simulink model "ssg_speader_r1"  (Simulink 7.6)
settings: Solver=ode45  StartTime=0.0  StopTime=128000  RelTol=1e-3
undefined symbols (not defined in the file): ROACH
libraries: xbsIndex_r4 x1066, xps_library x48, casper_library_misc x28, dspsigops x16, simulink x8
(part 1 of 11)
settings Model: Creator=mwagner  LastModifiedBy=mwagner
settings DebuggingCC: StrictBusMsg=Warning

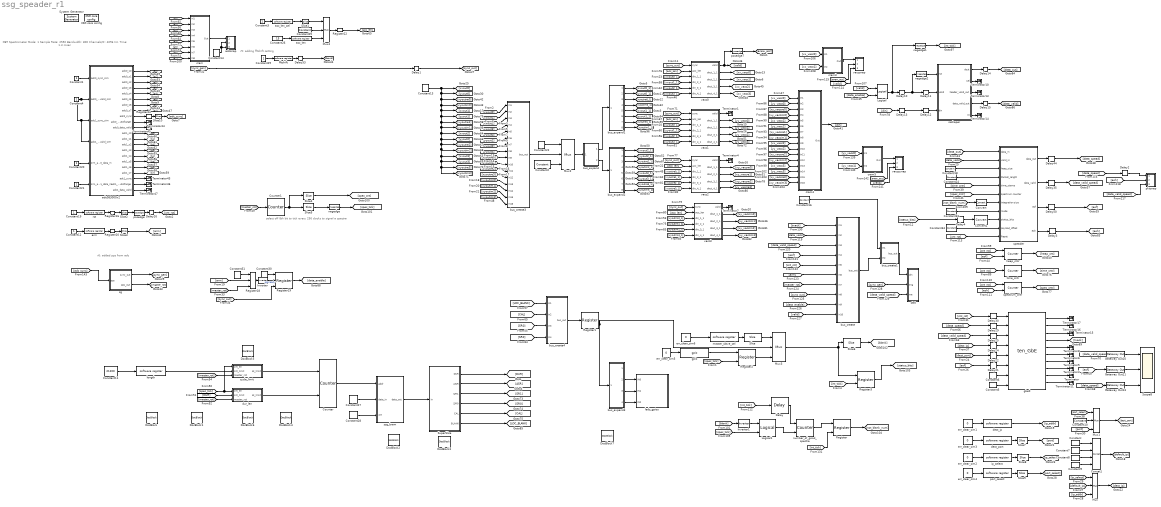
== system ssg_speader_r1 ==
  note: GBT Spectrometer
      | Mode: 1
      | Sample Rate: 2550
      | Bandwidth: 800
      | Channels/IF: 4096
      | Int. Time: 1.3 msec
  note: r5: adding fftshift setting
  note: r6: added pps from adc
  note: select off 8th bit to tick every 256 clocks to signal a spectra
  " System Generator" : xbsIndex_r4/ System Generator  Tag=genX  SystemSampleTime=-1  xilinxfamily=virtex5  part=xc5vsx95t  speed=-1  package=ff1136  synthesis_tool=XST  clock_wrapper=Clock Enables  directory=./vegas01_4tap_1024ch_220_r5a/sysgen  proj_type=Project Navigator  Synth_file=XST Defaults  Impl_file=ISE Defaults  testbench=off  simulink_period=1  sysclk_period=6.6667  dcm_input_clock_period=100  incr_netlist=off  trim_vbits=Everywhere in SubSystem  dbl_ovrd=According to Block Masks  core_generation=According to Block Masks  run_coregen=off  deprecated_control=off  eval_field=0  block_type=sysgen
      settings: block_version=10.1.3
  Concat1 : xbsIndex_r4/Concat  num_inputs=4  dbl_ovrd=off  block_type=concat
  Constant : xbsIndex_r4/Constant  const=10  gui_display_data_type=Fixed-point  arith_type=Unsigned  n_bits=8  bin_pt=0  preci_type=Single  exp_width=8  frac_width=24  explicit_period=on  period=1  equ=P=C  opselect=C  inp2=PCIN>>17  opr=+  inp1=P  carry=CIN  dbl_ovrd=off  block_type=constant
      settings: block_version=11.4
  Constant{1,4,20..21} (4 alike) : Constant  SampleTime=1
  Constant10 : xbsIndex_r4/Constant  const=10145  gui_display_data_type=Fixed-point  arith_type=Unsigned  n_bits=32  bin_pt=0  preci_type=Single  exp_width=8  frac_width=24  explicit_period=on  period=1  equ=P=C  opselect=C  inp2=PCIN>>17  opr=+  inp1=P  carry=CIN  dbl_ovrd=off  block_type=constant
  Constant11 : Constant  Value=21200  VectorParams1D=off
  Constant{3,12,19,29} (4 alike) : Constant
  Constant13 : xbsIndex_r4/Constant  const=1  gui_display_data_type=Fixed-point  arith_type=Unsigned  n_bits=32  bin_pt=0  preci_type=Single  exp_width=8  frac_width=24  explicit_period=on  period=1  equ=P=C  opselect=C  inp2=PCIN>>17  opr=+  inp1=P  carry=CIN  dbl_ovrd=off  block_type=constant
      settings: block_version=11.4
  Constant14 : xbsIndex_r4/Constant  const=1  gui_display_data_type=Fixed-point  arith_type=Boolean  n_bits=16  bin_pt=0  preci_type=Single  exp_width=8  frac_width=24  explicit_period=on  period=1  equ=P=C  opselect=C  inp2=PCIN>>17  opr=+  inp1=P  carry=CIN  dbl_ovrd=off  block_type=constant
      settings: block_version=11.4
  Constant16 : xbsIndex_r4/Constant  const=0  gui_display_data_type=Fixed-point  arith_type=Unsigned  n_bits=32-10  bin_pt=0  preci_type=Single  exp_width=8  frac_width=24  explicit_period=on  period=1  equ=P=C  opselect=C  inp2=PCIN>>17  opr=+  inp1=P  carry=CIN  dbl_ovrd=off  block_type=constant
  Constant18 : xbsIndex_r4/Constant  const=16384+8*6  gui_display_data_type=Fixed-point  arith_type=Unsigned  n_bits=40  bin_pt=0  preci_type=Single  exp_width=8  frac_width=24  explicit_period=on  period=1  equ=P=C  opselect=C  inp2=PCIN>>17  opr=+  inp1=P  carry=CIN  dbl_ovrd=off  block_type=constant
  Constant2 : xbsIndex_r4/Constant  const=0  gui_display_data_type=Fixed-point  arith_type=Unsigned  n_bits=512  bin_pt=0  preci_type=Single  exp_width=8  frac_width=24  explicit_period=on  period=1  equ=P=C  opselect=C  inp2=PCIN>>17  opr=+  inp1=P  carry=CIN  dbl_ovrd=off  block_type=constant
  Constant22 : xbsIndex_r4/Constant  const=0  gui_display_data_type=Boolean  arith_type=Boolean  n_bits=16  bin_pt=0  preci_type=Single  exp_width=8  frac_width=24  explicit_period=on  period=1  equ=P=C  opselect=C  inp2=PCIN>>17  opr=+  inp1=P  carry=CIN  dbl_ovrd=off  block_type=constant
      settings: block_version=11.4
  Constant24 : xbsIndex_r4/Constant  const=8192  gui_display_data_type=Fixed-point  arith_type=Unsigned  n_bits=40  bin_pt=0  preci_type=Single  exp_width=8  frac_width=24  explicit_period=on  period=1  equ=P=C  opselect=C  inp2=PCIN>>17  opr=+  inp1=P  carry=CIN  dbl_ovrd=off  block_type=constant
  Constant25 : xbsIndex_r4/Constant  const=63  gui_display_data_type=Fixed-point  arith_type=Unsigned  n_bits=32  bin_pt=0  preci_type=Single  exp_width=8  frac_width=24  explicit_period=on  period=1  equ=P=C  opselect=C  inp2=PCIN>>17  opr=+  inp1=P  carry=CIN  dbl_ovrd=off  block_type=constant
  Constant26 : Constant  Value=15
  Constant27 : xbsIndex_r4/Constant  const=0  gui_display_data_type=Fixed-point  arith_type=Unsigned  n_bits=32  bin_pt=0  preci_type=Single  exp_width=8  frac_width=24  explicit_period=on  period=1  equ=P=C  opselect=C  inp2=PCIN>>17  opr=+  inp1=P  carry=CIN  dbl_ovrd=off  block_type=constant
      settings: block_version=11.3
  Constant28 : xbsIndex_r4/Constant  const=0  gui_display_data_type=Fixed-point  arith_type=Boolean  n_bits=32  bin_pt=0  preci_type=Single  exp_width=8  frac_width=24  explicit_period=on  period=1  equ=P=C  opselect=C  inp2=PCIN>>17  opr=+  inp1=P  carry=CIN  dbl_ovrd=off  block_type=constant
      settings: block_version=11.3
  Constant30 : xbsIndex_r4/Constant  const=1  gui_display_data_type=Fixed-point  arith_type=Boolean  n_bits=16  bin_pt=0  preci_type=Single  exp_width=8  frac_width=24  explicit_period=on  period=1  equ=P=C  opselect=C  inp2=PCIN>>17  opr=+  inp1=P  carry=CIN  dbl_ovrd=off  block_type=constant
      settings: block_version=11.4
  Constant31 : xbsIndex_r4/Constant  const=1  gui_display_data_type=Fixed-point  arith_type=Boolean  n_bits=16  bin_pt=0  preci_type=Single  exp_width=8  frac_width=24  explicit_period=on  period=1  equ=P=C  opselect=C  inp2=PCIN>>17  opr=+  inp1=P  carry=CIN  dbl_ovrd=off  block_type=constant
      settings: block_version=11.4
  Constant33 : xbsIndex_r4/Constant  const=1  gui_display_data_type=Fixed-point  arith_type=Unsigned  n_bits=40  bin_pt=0  preci_type=Single  exp_width=8  frac_width=24  explicit_period=on  period=1  equ=P=C  opselect=C  inp2=PCIN>>17  opr=+  inp1=P  carry=CIN  dbl_ovrd=off  block_type=constant
  Constant34 : xbsIndex_r4/Constant  const=0  gui_display_data_type=Fixed-point  arith_type=Unsigned  n_bits=40  bin_pt=0  preci_type=Single  exp_width=8  frac_width=24  explicit_period=on  period=1  equ=P=C  opselect=C  inp2=PCIN>>17  opr=+  inp1=P  carry=CIN  dbl_ovrd=off  block_type=constant
  Constant5 : xbsIndex_r4/Constant  const=0  gui_display_data_type=Fixed-point  arith_type=Boolean  n_bits=1  bin_pt=0  preci_type=Single  exp_width=8  frac_width=24  explicit_period=on  period=1  equ=P=C  opselect=C  inp2=PCIN>>17  opr=+  inp1=P  carry=CIN  dbl_ovrd=off  block_type=constant
  Constant6 : xbsIndex_r4/Constant  const=0  gui_display_data_type=Fixed-point  arith_type=Boolean  n_bits=1  bin_pt=0  preci_type=Single  exp_width=8  frac_width=24  explicit_period=on  period=1  equ=P=C  opselect=C  inp2=PCIN>>17  opr=+  inp1=P  carry=CIN  dbl_ovrd=off  block_type=constant
  Constant7 : xbsIndex_r4/Constant  const=0  gui_display_data_type=Fixed-point  arith_type=Unsigned  n_bits=8  bin_pt=0  preci_type=Single  exp_width=8  frac_width=24  explicit_period=on  period=1  equ=P=C  opselect=C  inp2=PCIN>>17  opr=+  inp1=P  carry=CIN  dbl_ovrd=off  block_type=constant
      settings: block_version=11.4
  Constant8 : xbsIndex_r4/Constant  const=0  gui_display_data_type=Fixed-point  arith_type=Unsigned  n_bits=8  bin_pt=0  preci_type=Single  exp_width=8  frac_width=24  explicit_period=on  period=1  equ=P=C  opselect=C  inp2=PCIN>>17  opr=+  inp1=P  carry=CIN  dbl_ovrd=off  block_type=constant
      settings: block_version=11.4
  Constant9 : xbsIndex_r4/Constant  const=145  gui_display_data_type=Fixed-point  arith_type=Unsigned  n_bits=8  bin_pt=0  preci_type=Single  exp_width=8  frac_width=24  explicit_period=on  period=1  equ=P=C  opselect=C  inp2=PCIN>>17  opr=+  inp1=P  carry=CIN  dbl_ovrd=off  block_type=constant
      settings: block_version=11.4
  Convert : xbsIndex_r4/Convert  gui_display_data_type=Fixed-point  arith_type=Unsigned  n_bits=40  bin_pt=0  float_type=Single  exp_bits=8  fraction_bits=24  quantization=Truncate  overflow=Wrap  en=off  latency=0  dbl_ovrd=off  pipeline=off  block_type=convert
      settings: block_version=11.4
  Convert1 : xbsIndex_r4/Convert  gui_display_data_type=Fixed-point  arith_type=Unsigned  n_bits=40  bin_pt=0  float_type=Single  exp_bits=8  fraction_bits=24  quantization=Truncate  overflow=Wrap  en=off  latency=0  dbl_ovrd=off  pipeline=off  block_type=convert
  Counter : xbsIndex_r4/Counter  cnt_type=Free Running  cnt_to=Inf  operation=Up  start_count=0  cnt_by_val=1  arith_type=Unsigned  n_bits=8  bin_pt=0  load_pin=off  rst=on  en=on  explicit_period=on  period=1  dbl_ovrd=off  use_behavioral_HDL=off  implementation=DSP48  block_type=counter
      settings: block_version=11.3
  Counter1 : xbsIndex_r4/Counter  cnt_type=Free Running  cnt_to=Inf  operation=Up  start_count=0  cnt_by_val=1  arith_type=Unsigned  n_bits=48  bin_pt=0  load_pin=off  rst=on  en=off  explicit_period=on  period=1  dbl_ovrd=off  use_behavioral_HDL=off  implementation=DSP48  block_type=counter
      settings: block_version=11.3
  Delay : xbsIndex_r4/Delay  rst=off  infoeditControl=Selection of Reset will increase slice count due to use of real FFs and instead of SRLs  en=off  latency=1  dbl_ovrd=off  reg_retiming=off  block_type=delay
  Delay1 : xbsIndex_r4/Delay  rst=off  infoeditControl=Selection of Reset will increase slice count due to use of real FFs and instead of SRLs  en=off  latency=1000  dbl_ovrd=off  reg_retiming=off  block_type=delay
      settings: block_version=11.4
  Delay{10..13} (4 alike) : xbsIndex_r4/Delay  rst=off  infoeditControl=Selection of Reset will increase slice count due to use of real FFs and instead of SRLs  en=off  latency=2  dbl_ovrd=off  reg_retiming=on  block_type=delay
  Delay14 : xbsIndex_r4/Delay  rst=off  infoeditControl=Selection of Reset will increase slice count due to use of real FFs and instead of SRLs  en=off  latency=4  dbl_ovrd=off  reg_retiming=on  block_type=delay
  Delay15 : xbsIndex_r4/Delay  rst=off  infoeditControl=Selection of Reset will increase slice count due to use of real FFs and instead of SRLs  en=off  latency=4  dbl_ovrd=off  reg_retiming=on  block_type=delay
  Delay2 : xbsIndex_r4/Delay  rst=off  infoeditControl=Selection of Reset will increase slice count due to use of real FFs and instead of SRLs  en=off  latency=12  dbl_ovrd=off  reg_retiming=on  block_type=delay
  Delay{3..4,21..22,24..25,29..30,35,44,50} (11 alike) : xbsIndex_r4/Delay  rst=off  infoeditControl=Selection of Reset will increase slice count due to use of real FFs and instead of SRLs  en=off  latency=1  dbl_ovrd=off  reg_retiming=on  block_type=delay
  Delay26 : xbsIndex_r4/Delay  rst=off  infoeditControl=Selection of Reset will increase slice count due to use of real FFs and instead of SRLs  en=off  latency=8  dbl_ovrd=off  reg_retiming=on  block_type=delay
  Delay53 : xbsIndex_r4/Delay  rst=off  infoeditControl=Selection of Reset will increase slice count due to use of real FFs and instead of SRLs  en=off  latency=1  dbl_ovrd=off  reg_retiming=off  block_type=delay
      settings: block_version=11.4
  DocBlock{,1..7} (8 alike) : simulink/Model-Wide Utilities/DocBlock  SystemSampleTime=-1  DocumentType=Text
  Gateway Out10 : xbsIndex_r4/Gateway Out  hdl_port=on  timing_constraint=None  locs_specified=off  LOCs={}  block_type=gatewayout
      settings: infoedit="Gateway out block.  Converts Xilinx fixed point inputs into ouputs of type Simulink integer, double, or fixed point.<br><br>Hardware notes:  In hardware these blocks become top level output ports or are discarded, depending on how they are configured."  block_version=11.4
  Gateway Out11 : xbsIndex_r4/Gateway Out  hdl_port=on  timing_constraint=None  locs_specified=off  LOCs={}  block_type=gatewayout
      settings: infoedit="Gateway out block.  Converts Xilinx fixed point inputs into ouputs of type Simulink integer, double, or fixed point.<br><br>Hardware notes:  In hardware these blocks become top level output ports or are discarded, depending on how they are configured."  block_version=11.4
  Gateway Out13 : xbsIndex_r4/Gateway Out  hdl_port=on  timing_constraint=None  locs_specified=off  LOCs={}  block_type=gatewayout
      settings: infoedit="Gateway out block.  Converts Xilinx fixed point inputs into ouputs of type Simulink integer, double, or fixed point.<br><br>Hardware notes:  In hardware these blocks become top level output ports or are discarded, depending on how they are configured."  block_version=11.4
  Inverter : xbsIndex_r4/Inverter  en=off  latency=0  dbl_ovrd=off  block_type=inv
      settings: block_version=11.4
  Inverter1 : xbsIndex_r4/Inverter  en=off  latency=0  dbl_ovrd=off  block_type=inv
  Logical : xbsIndex_r4/Logical  logical_function=AND  inputs=2  en=off  latency=0  precision=Full  arith_type=Unsigned  n_bits=16  bin_pt=0  align_bp=on  dbl_ovrd=off  block_type=logical
      settings: block_version=11.4
  Logical1 : xbsIndex_r4/Logical  logical_function=AND  inputs=2  en=off  latency=0  precision=Full  arith_type=Unsigned  n_bits=16  bin_pt=0  align_bp=on  dbl_ovrd=off  block_type=logical
  Mux{,1..2,4} (4 alike) : xbsIndex_r4/Mux  inputs=2  en=off  latency=1  precision=Full  arith_type=Unsigned  n_bits=16  bin_pt=14  quantization=Truncate  overflow=Wrap  dbl_ovrd=off  block_type=mux
      Mux settings: block_version=11.4
      Mux1 settings: block_version=11.4
      Mux4 settings: block_version=11.4
  Mux3 : xbsIndex_r4/Mux  inputs=2  en=off  latency=0  precision=Full  arith_type=Unsigned  n_bits=16  bin_pt=14  quantization=Truncate  overflow=Wrap  dbl_ovrd=off  block_type=mux
  Register : xbsIndex_r4/Register  init=0  rst=off  en=on  dbl_ovrd=off  block_type=register
  Register{1,16,20,22,44} (5 alike) : xbsIndex_r4/Register  init=0  rst=off  en=off  dbl_ovrd=off  block_type=register
      settings: block_version=11.4
  Register18 : xbsIndex_r4/Register  init=0  rst=on  en=on  dbl_ovrd=off  block_type=register
      settings: block_version=11.4
  Register19 : xbsIndex_r4/Register  init=0  rst=on  en=on  dbl_ovrd=off  block_type=register
      settings: block_version=11.4
  Register2 : xbsIndex_r4/Register  init=0  rst=off  en=on  dbl_ovrd=off  block_type=register
      settings: block_version=11.4
  Register3 : xbsIndex_r4/Register  init=0  rst=off  en=on  dbl_ovrd=off  block_type=register
      settings: block_version=11.4
  Scope8 : Scope  NumInputPorts=3
      settings: TimeRange=4500  YMin=0~-1~0  YMax=1~1~1.75e+13  SaveName=ScopeData8  MaxDataPoints=100000
  Slice{,1..3,8..10} (7 alike) : xbsIndex_r4/Slice  nbits=1  boolean_output=on  mode=Lower Bit Location + Width  bit1=0  base1=MSB of Input  bit0=0  base0=LSB of Input  dbl_ovrd=off  block_type=slice
      Slice1 settings: block_version=10.1.3
      Slice10 settings: infoedit="Extracts a given range of bits from each input sample and presents it at the output.  The output type is ordinarily unsigned with binary point at zero, but can be Boolean when the slice is one bit wide.<P><P>Hardware notes: In hardware this block costs nothing."  block_version=10.1.3
      Slice2 settings: block_version=10.1.3
      Slice3 settings: block_version=10.1.3
      Slice8 settings: block_version=10.1.3
      Slice9 settings: block_version=10.1.3
  Slice4 : xbsIndex_r4/Slice  nbits=40  boolean_output=off  mode=Lower Bit Location + Width  bit1=0  base1=MSB of Input  bit0=8  base0=LSB of Input  dbl_ovrd=off  block_type=slice
      settings: block_version=10.1.3
  Slice5 : xbsIndex_r4/Slice  nbits=1  boolean_output=on  mode=Lower Bit Location + Width  bit1=7  base1=MSB of Input  bit0=7  base0=LSB of Input  dbl_ovrd=off  block_type=slice
      settings: block_version=10.1.3
  Slice6 : xbsIndex_r4/Slice  nbits=1  boolean_output=on  mode=Upper Bit Location + Width  bit1=0  base1=MSB of Input  bit0=0  base0=LSB of Input  dbl_ovrd=off  block_type=slice
  Slice7 : xbsIndex_r4/Slice  nbits=16  boolean_output=off  mode=Lower Bit Location + Width  bit1=0  base1=MSB of Input  bit0=0  base0=LSB of Input  dbl_ovrd=off  block_type=slice
      settings: infoedit="Extracts a given range of bits from each input sample and presents it at the output.  The output type is ordinarily unsigned with binary point at zero, but can be Boolean when the slice is one bit wide.<P><P>Hardware notes: In hardware this block costs nothing."  block_version=10.1.3
  SuperSlice : Subsystem  AncestorBlock=gavrt_library/SuperSlice  mask(superslice){slices=[27,1,1,1,1,1]}
      mask prompts: slices "Slice pattern"
      mask help:
      | Slices the input word into consecutive outputs of arbitrary width.
      | Slice pattern should be a vector with each entry representing the width of that particular slice. The first entry is the MSB slice and the last is the LSB slice.
      | If a slice is given width -1, that slice will have a boolean output.
      | Ex: -1*ones(1,32)  -- Slice a 32 bit word into seperate boolean flags
      | [16, 8, -1*ones(1,8)] -- Slice a 32 bit word into the MSW, a byte, and the least significant 8 bits
      mask init:
      | superslice_init(gcb, 'slices', slices);
  Terminator{,1,3..8,10..11,13..17,43..47} (20 alike) : Terminator
  XSG core config : xps_library/XSG core config  Tag=xps:xsg  SystemSampleTime=-1  hw_sys=ROACH:sx95t  ibob_linux=off  clk_src=adc0_clk  iBOB_clk_src=adc0_clk  BEE2_ctrl_clk_src=sys_clk  BEE2_usr_clk_src=sys_clk  ROACH_clk_src=adc0_clk  ROACH2_clk_src=adc0_clk  CORR_clk_src=sys_clk  gpio_clk_io_group=iBOB:sma  gpio_clk_bit_index=0  clk_rate=150  sample_period=1  synthesis_tool=XST  mpc_type=powerpc440_ext
  acc_len : xps_library/software register  Tag=xps:sw_reg  SystemSampleTime=-1  io_dir=From Processor  arith_type=Unsigned  bitwidth=32  bin_pt=0  sample_period=1  gw_name=ssg_speader_crash_acc_len_user_data_out
      link override convert: arith_type=Unsigned  n_bits=32  bin_pt=0
      link override r_spec_2048_r102_cnt_rst_user_data_out: arith_type=Unsigned  n_bits=32  bin_pt=0  period=1
      link override r_spec_2048_r102_nosim_cnt_rst_user_data_out: arith_type=Unsigned  n_bits=32  bin_pt=0  period=1
      link override r_spec_2048_r103_cnt_rst_user_data_out: arith_type=Unsigned  n_bits=32  bin_pt=0  period=1
      link override roach_spec_no10gbe_sync_cnt_rst_user_data_out: arith_type=Unsigned  n_bits=32  bin_pt=0  period=1
      link override roach_spec_rst_cnt_user_data_out: arith_type=Unsigned  n_bits=32  bin_pt=0  period=1
      link override roach_spec_rst_sync_cnt_user_data_out: arith_type=Unsigned  n_bits=32  bin_pt=0  period=1
  acc_len_sel : xps_library/software register  Tag=xps:sw_reg  SystemSampleTime=-1  io_dir=From Processor  arith_type=Unsigned  bitwidth=32  bin_pt=0  sample_period=1  gw_name=ssg_speader_crash_acc_len_sel_user_data_out
      link override convert: arith_type=Unsigned  n_bits=32  bin_pt=0
      link override r_spec_2048_r102_cnt_rst_user_data_out: arith_type=Unsigned  n_bits=32  bin_pt=0  period=1
      link override r_spec_2048_r102_nosim_cnt_rst_user_data_out: arith_type=Unsigned  n_bits=32  bin_pt=0  period=1
      link override r_spec_2048_r103_cnt_rst_user_data_out: arith_type=Unsigned  n_bits=32  bin_pt=0  period=1
      link override roach_spec_no10gbe_sync_cnt_rst_user_data_out: arith_type=Unsigned  n_bits=32  bin_pt=0  period=1
      link override roach_spec_rst_cnt_user_data_out: arith_type=Unsigned  n_bits=32  bin_pt=0  period=1
      link override roach_spec_rst_sync_cnt_user_data_out: arith_type=Unsigned  n_bits=32  bin_pt=0  period=1
  adc083000x2 : Subsystem  Tag=xps:adc083000x2  AncestorBlock=xps_library/adc083000x2  mask(adc_083000x2){use_adc0=on, use_adc1=on, demux_adc=off, clock_sync=off, verbose=off, using_ctrl=on, adc_clk_rate=600, sample_period=1, bit_width=8}
      mask prompts: use_adc0 "Use ZD0K0?"; use_adc1 "Use ZDOK1?"; demux_adc "Demux ADCs by 2?"; clock_sync "Interleave 2 ADC boards?"; verbose "Verbose Block Creation?"; using_ctrl "Add ports for control registers?"; adc_clk_rate "ADC clock rate (MHz)"; sample_period "Sample Period"; bit_width "Output Bit Width"
      mask help:
      | The ADC block converts analog inputs to digital outputs.
      | Every clock cycle, the inputs are sampled and digitized to
      | 8 bit binary point numbers in the range of [-1, 1).
      |
      | Online block-specific documentation: http://casper.berkeley.edu/wiki/Adc083000
      mask init:
      | adc083000_mask;
      mask Help: eval('xlWeb([getenv(''MLIB_ROOT''), ''\doc\html\sys_adc\sys_adc.html''])')
  adcsnap : Subsystem  AncestorBlock=casper_library_scopes/snap64  mask(snap64){nsamples=11}
      mask prompts: nsamples "No. of samples(2^?)"
      mask help:
      | The <i>snap</i> block provides a packaged solution to capturing data from
      | the FPGA fabric and making it accessible from the CPU.  The block comes in
      | 2 flavors: <i>snap</i> (which captures to a 32 bit wide Shared BRAM), and
      | <i>snap64</i> (which captures to 2x32 bit wide Shared BRAMs to effect a
      | 64 bit capture).
      mask Help: eval('xlWeb(''http://casper.berkeley.edu/wiki/Snap'')')
  arm : xps_library/software register  Tag=xps:sw_reg  SystemSampleTime=-1  io_dir=From Processor  arith_type=Unsigned  bitwidth=32  bin_pt=0  sample_period=1  gw_name=ssg_speader_crash_arm_user_data_out
      link override convert: arith_type=Unsigned  n_bits=32  bin_pt=0
      link override r_spec_2048_r102_cnt_rst_user_data_out: arith_type=Unsigned  n_bits=32  bin_pt=0  period=1
      link override r_spec_2048_r102_nosim_cnt_rst_user_data_out: arith_type=Unsigned  n_bits=32  bin_pt=0  period=1
      link override r_spec_2048_r103_cnt_rst_user_data_out: arith_type=Unsigned  n_bits=32  bin_pt=0  period=1
      link override roach_spec_no10gbe_sync_cnt_rst_user_data_out: arith_type=Unsigned  n_bits=32  bin_pt=0  period=1
      link override roach_spec_rst_cnt_user_data_out: arith_type=Unsigned  n_bits=32  bin_pt=0  period=1
      link override roach_spec_rst_sync_cnt_user_data_out: arith_type=Unsigned  n_bits=32  bin_pt=0  period=1
  bus_create : Subsystem  AncestorBlock=casper_library_flow_control/bus_create  mask(bus_create){inputNum=10}
      mask prompts: inputNum "Number of inputs:"
      mask init:
      | bus_create_init(gcb,...
      |     'inputNum', inputNum);
  bus_create1 : Subsystem  AncestorBlock=casper_library_flow_control/bus_create  mask(bus_create){inputNum=2}
      mask prompts: inputNum "Number of inputs:"
      mask init:
      | bus_create_init(gcb,...
      |     'inputNum', inputNum);
  bus_create3 : Subsystem  AncestorBlock=casper_library_flow_control/bus_create  mask(bus_create){inputNum=16}
      mask prompts: inputNum "Number of inputs:"
      mask init:
      | bus_create_init(gcb,...
      |     'inputNum', inputNum);
  bus_create4 : Subsystem  AncestorBlock=casper_library_flow_control/bus_create  mask(bus_create){inputNum=4}
      mask prompts: inputNum "Number of inputs:"
      mask init:
      | bus_create_init(gcb,...
      |     'inputNum', inputNum);
  bus_expand : Subsystem  AncestorBlock=casper_library_flow_control/bus_expand  mask(bus_expand){mode=divisions of equal size, outputNum=2, outputWidth=256, outputBinaryPt=0, outputArithmeticType=0, outputToWorkspace=off, variablePrefix=out, outputToModelAsWell=on}
      mask prompts: outputNum "Number of outputs:"; outputWidth "Output width:"; outputBinaryPt "Output binary point position:"; outputArithmeticType "Output arithmetic type: (Unsigned=0, Signed=1, Boolean=2)"; outputToWorkspace "Output to workspace?"; variablePrefix "Variable name prefix:"; outputToModelAsWell "Output to model as well?"
      mask help:
      | Expands a 'bus' made using a bus_create or Xilinx
      | concat block.
      | The input will be divided into the specified number
      | of outputs with the specified arithmetic types.
      | Divisions are made from most significant bit.
      mask init:
      | bus_expand_init(gcb,...
      |     'mode', mode, ...
      |     'outputNum', outputNum, ...
      |     'outputWidth', outputWidth, ...
      |     'outputBinaryPt', outputBinaryPt, ...
      |     'outputArithmeticType', outputArithmeticType, ...
      |     'outputToWorkspace', outputToWorkspace, ...
      |     'variablePrefix', variablePrefix, ...
      |     'outputToModelAsWell', outputToModelAsWell);
      settings: AttributesFormatString=2 outputs
      mask StyleString: popup(divisions of equal size|divisions of arbitrary size),edit,edit,edit,edit,checkbox,edit,checkbox
      mask CallbackString: bus_expand_callback();||bus_expand_callback();|||bus_expand_callback();||
  bus_expand1 : Subsystem  AncestorBlock=casper_library_flow_control/bus_expand  mask(bus_expand){mode=divisions of equal size, outputNum=8, outputWidth=32, outputBinaryPt=31, outputArithmeticType=0, outputToWorkspace=off, variablePrefix=out, outputToModelAsWell=on}
      mask prompts: outputNum "Number of outputs:"; outputWidth "Output width:"; outputBinaryPt "Output binary point position:"; outputArithmeticType "Output arithmetic type: (Unsigned=0, Signed=1, Boolean=2)"; outputToWorkspace "Output to workspace?"; variablePrefix "Variable name prefix:"; outputToModelAsWell "Output to model as well?"
      mask help:
      | Expands a 'bus' made using a bus_create or Xilinx
      | concat block.
      | The input will be divided into the specified number
      | of outputs with the specified arithmetic types.
      | Divisions are made from most significant bit.
      mask init: same as ssg_speader_r1/bus_expand
      settings: AttributesFormatString=8 outputs
      mask StyleString: popup(divisions of equal size|divisions of arbitrary size),edit,edit,edit,edit,checkbox,edit,checkbox
      mask CallbackString: bus_expand_callback();||bus_expand_callback();|||bus_expand_callback();||
  bus_expand2 : Subsystem  AncestorBlock=casper_library_flow_control/bus_expand  mask(bus_expand){mode=divisions of equal size, outputNum=8, outputWidth=32, outputBinaryPt=31, outputArithmeticType=1, outputToWorkspace=off, variablePrefix=out, outputToModelAsWell=on}
      mask prompts: outputNum "Number of outputs:"; outputWidth "Output width:"; outputBinaryPt "Output binary point position:"; outputArithmeticType "Output arithmetic type: (Unsigned=0, Signed=1, Boolean=2)"; outputToWorkspace "Output to workspace?"; variablePrefix "Variable name prefix:"; outputToModelAsWell "Output to model as well?"
      mask help:
      | Expands a 'bus' made using a bus_create or Xilinx
      | concat block.
      | The input will be divided into the specified number
      | of outputs with the specified arithmetic types.
      | Divisions are made from most significant bit.
      mask init: same as ssg_speader_r1/bus_expand
      settings: AttributesFormatString=8 outputs
      mask StyleString: popup(divisions of equal size|divisions of arbitrary size),edit,edit,edit,edit,checkbox,edit,checkbox
      mask CallbackString: bus_expand_callback();||bus_expand_callback();|||bus_expand_callback();||
  bus_expand3 : Subsystem  AncestorBlock=casper_library_flow_control/bus_expand  mask(bus_expand){mode=divisions of equal size, outputNum=4, outputWidth=1, outputBinaryPt=0, outputArithmeticType=2, outputToWorkspace=off, variablePrefix=out, outputToModelAsWell=on}
      mask prompts: outputNum "Number of outputs:"; outputWidth "Output width:"; outputBinaryPt "Output binary point position:"; outputArithmeticType "Output arithmetic type: (Unsigned=0, Signed=1, Boolean=2)"; outputToWorkspace "Output to workspace?"; variablePrefix "Variable name prefix:"; outputToModelAsWell "Output to model as well?"
      mask help:
      | Expands a 'bus' made using a bus_create or Xilinx
      | concat block.
      | The input will be divided into the specified number
      | of outputs with the specified arithmetic types.
      | Divisions are made from most significant bit.
      mask init: same as ssg_speader_r1/bus_expand
      settings: AttributesFormatString=4 outputs
      mask StyleString: popup(divisions of equal size|divisions of arbitrary size),edit,edit,edit,edit,checkbox,edit,checkbox
      mask CallbackString: bus_expand_callback();||bus_expand_callback();|||bus_expand_callback();||
  cram : Subsystem  AncestorBlock=gavrt_library/cram  mask(cram){num_slice=8}
      mask prompts: num_slice "Number of slices"
      mask help: Concatenates inputs together after forcing binary point to zero.
      mask init:
      | cram_init(gcb, ...
      |     'num_slice', num_slice);
  cram3 : Subsystem  AncestorBlock=gavrt_library/cram  mask(cram){num_slice=2}
      mask prompts: num_slice "Number of slices"
      mask help: Concatenates inputs together after forcing binary point to zero.
      mask init:
      | cram_init(gcb, ...
      |     'num_slice', num_slice);
  cram4 : Subsystem  AncestorBlock=gavrt_library/cram  mask(cram){num_slice=16}
      mask prompts: num_slice "Number of slices"
      mask help: Concatenates inputs together after forcing binary point to zero.
      mask init:
      | cram_init(gcb, ...
      |     'num_slice', num_slice);
  cram5 : Subsystem  AncestorBlock=gavrt_library/cram  mask(cram){num_slice=2}
      mask prompts: num_slice "Number of slices"
      mask help: Concatenates inputs together after forcing binary point to zero.
      mask init:
      | cram_init(gcb, ...
      |     'num_slice', num_slice);
  cycle_limit : Subsystem
  dest_ip : xps_library/software register  Tag=xps:sw_reg  SystemSampleTime=-1  io_dir=From Processor  arith_type=Unsigned  bitwidth=32  bin_pt=0  sample_period=1  gw_name=ssg_speader_crash_dest_ip_user_data_out
      link override r_10gbe_demo_dest_ip_user_data_out: arith_type=Unsigned  n_bits=32  bin_pt=0  period=1
      link override r_10gbe_test_dest_ip_user_data_out: arith_type=Unsigned  n_bits=32  bin_pt=0  period=1
      link override r_xaui_test_cnt_rst_user_data_out: arith_type=Unsigned  n_bits=32  bin_pt=0  period=1
  dest_port : xps_library/software register  Tag=xps:sw_reg  SystemSampleTime=-1  io_dir=From Processor  arith_type=Unsigned  bitwidth=32  bin_pt=0  sample_period=1  gw_name=ssg_speader_crash_dest_port_user_data_out
      link override r_10gbe_demo_dest_port_user_data_out: arith_type=Unsigned  n_bits=32  bin_pt=0  period=1
      link override r_10gbe_test_dest_port_user_data_out: arith_type=Unsigned  n_bits=32  bin_pt=0  period=1
      link override r_xaui_test_cnt_rst_user_data_out: arith_type=Unsigned  n_bits=32  bin_pt=0  period=1
  dur_len : Subsystem
  err_clear_sim{1..6} (6 alike) : Constant  Value=0
  fftshift : xps_library/software register  Tag=xps:sw_reg  SystemSampleTime=-1  io_dir=From Processor  arith_type=Unsigned  bitwidth=32  bin_pt=0  sample_period=1  gw_name=ssg_speader_crash_fftshift_user_data_out
  gbe0 : xps_library/ten_GbE  Tag=xps:tengbe  SystemSampleTime=-1  port=ROACH:0  mac_lite=off  open_phy=off  show_param=off  pre_emph=3  swing=800  fab_en=off  fab_mac=0  fab_ip=0  fab_udp=0  fab_gate=0
  gpio : xps_library/gpio  Tag=xps:gpio  SystemSampleTime=-1  io_group=ROACH:gpiob  io_dir=in  arith_type=Unsigned  bitwidth=4  bin_pt=0  bit_index=[1:4]  sample_period=1  use_single_ended=off  use_ddr=off  reg_iob=on  reg_clk_phase=0  termination=None
  heap_cntr : xbsIndex_r4/Counter  cnt_type=Free Running  cnt_to=Inf  operation=Up  start_count=0  cnt_by_val=1  arith_type=Unsigned  n_bits=40  bin_pt=0  load_pin=off  rst=on  en=on  explicit_period=on  period=1  dbl_ovrd=off  use_behavioral_HDL=off  implementation=Fabric  block_type=counter
      settings: block_version=11.4
  ip_select : xps_library/software register  Tag=xps:sw_reg  SystemSampleTime=-1  io_dir=From Processor  arith_type=Unsigned  bitwidth=32  bin_pt=0  sample_period=1  gw_name=ssg_speader_crash_ip_select_user_data_out
      link override r_10gbe_demo_gbe_core_rst_user_data_out: arith_type=Unsigned  n_bits=32  bin_pt=0  period=1
      link override r_10gbe_test_cnt_rst_user_data_out: arith_type=Unsigned  n_bits=32  bin_pt=0  period=1
      link override r_10gbe_test_gbe_core_rst_user_data_out: arith_type=Unsigned  n_bits=32  bin_pt=0  period=1
      link override r_xaui_test_cnt_rst_user_data_out: arith_type=Unsigned  n_bits=32  bin_pt=0  period=1
  leds_gpios : Subsystem
  length : xps_library/software register  Tag=xps:sw_reg  SystemSampleTime=-1  io_dir=From Processor  arith_type=Unsigned  bitwidth=32  bin_pt=0  sample_period=1  gw_name=ssg_speader_crash_length_user_data_out
  master_slave_sel : xps_library/software register  Tag=xps:sw_reg  SystemSampleTime=-1  io_dir=From Processor  arith_type=Unsigned  bitwidth=32  bin_pt=0  sample_period=1  gw_name=ssg_speader_crash_master_slave_sel_user_data_out
  negedge : casper_library_misc/negedge  Tag=Rising Edge Detector  SystemSampleTime=-1
  negedge1 : casper_library_misc/negedge  Tag=Rising Edge Detector  SystemSampleTime=-1
  negedge2 : casper_library_misc/negedge  Tag=Rising Edge Detector  SystemSampleTime=-1
  number_of_good_spectra : xbsIndex_r4/Counter  cnt_type=Free Running  cnt_to=Inf  operation=Up  start_count=0  cnt_by_val=1  arith_type=Unsigned  n_bits=16  bin_pt=0  load_pin=off  rst=on  en=on  explicit_period=on  period=1  dbl_ovrd=off  use_behavioral_HDL=off  implementation=Fabric  block_type=counter
  pktsnap : Subsystem  AncestorBlock=casper_library_scopes/snap64  mask(snap64){nsamples=11}
      mask prompts: nsamples "No. of samples(2^?)"
      mask help:
      | The <i>snap</i> block provides a packaged solution to capturing data from
      | the FPGA fabric and making it accessible from the CPU.  The block comes in
      | 2 flavors: <i>snap</i> (which captures to a 32 bit wide Shared BRAM), and
      | <i>snap64</i> (which captures to 2x32 bit wide Shared BRAMs to effect a
      | 64 bit capture).
      mask Help: eval('xlWeb(''http://casper.berkeley.edu/wiki/Snap'')')
  port_select : xps_library/software register  Tag=xps:sw_reg  SystemSampleTime=-1  io_dir=From Processor  arith_type=Unsigned  bitwidth=32  bin_pt=0  sample_period=1  gw_name=ssg_speader_crash_port_select_user_data_out
      link override r_10gbe_demo_gbe_core_rst_user_data_out: arith_type=Unsigned  n_bits=32  bin_pt=0  period=1
      link override r_10gbe_test_cnt_rst_user_data_out: arith_type=Unsigned  n_bits=32  bin_pt=0  period=1
      link override r_10gbe_test_gbe_core_rst_user_data_out: arith_type=Unsigned  n_bits=32  bin_pt=0  period=1
      link override r_xaui_test_cnt_rst_user_data_out: arith_type=Unsigned  n_bits=32  bin_pt=0  period=1
  posedge : casper_library_misc/posedge  Tag=Rising Edge Detector  SystemSampleTime=-1
  posedge7 : casper_library_misc/posedge  Tag=Rising Edge Detector  SystemSampleTime=-1
  reshaper : Subsystem  mask{inwid=512, inlen=256, outwid=64, outchunk=1024, headlen=10}
      mask prompts: inwid "Input Width (bits)"; inlen "Input Length (clocks)"; outwid "Output Width (bits)"; outchunk "Output Chunk Length (clocks)"; headlen "Header Length"
      mask help:
      | This block takes wide input data and reshapes it to a narrower (or the same)
      | bit width, and breaks it into packets, between which a header can be inserted.
      | Each input data frame must be proceeded by a reset pulse. The input data can be
      | disjoint, with a pulsed valid signal. When the reset signal is pulsed, the previous data
      | frame will be read out. Therefore the number of clocks to read out the header and
      | data must be greater than the number of clocks between two frames (rst signals).
      |
      | The sel signal can be used to drive the select input of a mux which muxes between
      | the data stream (dout) and the indicated number of header words. The header_valid_out
      | signal goes high for each word of the header. dout should be connected to input
      | 0 of the mux. The data_valid_out goes high for each output data value. The st output
      | is for debug access to the internal state machine state.
      mask init:
      | l2inlen = ceil(log2(inlen))
      | l2outchunk = ceil(log2(outchunk))
      | outlen = inlen*(inwid/outwid)
      | nchunk = outlen/outchunk
      | l2headlen = ceil(log2(headlen))
      | l2outlen = ceil(log2(outlen))
  rst : xps_library/software register  Tag=xps:sw_reg  SystemSampleTime=-1  io_dir=From Processor  arith_type=Unsigned  bitwidth=32  bin_pt=0  sample_period=1  gw_name=ssg_speader_crash_rst_user_data_out
      link override convert: arith_type=Unsigned  n_bits=32  bin_pt=0
      link override r_spec_2048_r102_cnt_rst_user_data_out: arith_type=Unsigned  n_bits=32  bin_pt=0  period=1
      link override r_spec_2048_r102_nosim_cnt_rst_user_data_out: arith_type=Unsigned  n_bits=32  bin_pt=0  period=1
      link override r_spec_2048_r103_cnt_rst_user_data_out: arith_type=Unsigned  n_bits=32  bin_pt=0  period=1
      link override roach_spec_no10gbe_sync_cnt_rst_user_data_out: arith_type=Unsigned  n_bits=32  bin_pt=0  period=1
      link override roach_spec_rst_cnt_user_data_out: arith_type=Unsigned  n_bits=32  bin_pt=0  period=1
      link override roach_spec_rst_sync_cnt_user_data_out: arith_type=Unsigned  n_bits=32  bin_pt=0  period=1
  sg : Subsystem
  speader : Subsystem  AncestorBlock=gbt_library/speader  mask{spead_msw=64, spead_lsw=40, num_items=6, num_payloads=2}
      mask prompts: num_items "Number of items (+5)"; num_payloads "number of payloads"
      mask help:
      | The size of the heap and payload are in Bytes.
      | If there is one packet per heap then payload_offset is 0.
      | All the input must be not longer than 40 bits.
  spectrum_cntr : xbsIndex_r4/Counter  cnt_type=Free Running  cnt_to=Inf  operation=Up  start_count=0  cnt_by_val=1  arith_type=Unsigned  n_bits=40  bin_pt=0  load_pin=off  rst=on  en=on  explicit_period=on  period=1  dbl_ovrd=off  use_behavioral_HDL=off  implementation=Fabric  block_type=counter
      settings: block_version=11.4
  ssg_bram : Subsystem  Tag=xps:bram  AncestorBlock=xps_library/Shared BRAM  mask{arith_type=Unsigned, addr_width=11, data_width=32, data_bin_pt=0, init_vals=[12801,121600,3201,3203,57602,3203,3201,121600,12801,12805,121604,3205,3207,57606,3207,3205,121604,12805,0:0], sample_rate=1}
      mask prompts: arith_type "Output Data Type"; addr_width "Address width"; data_width "Data Width"; data_bin_pt "Data Binary Point"; init_vals "Initial 32-bit values (simulation only)"; sample_rate "Sample rate"
      mask init:
      | shared_bram_mask;
      mask StyleString: popup(Unsigned|Signed  (2's comp)),edit,popup(8|16|32|64|128),edit,edit,edit
  stat : Subsystem  AncestorBlock=casper_library_scopes/snap  mask(snap){nsamples=13}
      mask prompts: nsamples "No. of samples(2^?)"
      mask help:
      | The <i>snap</i> block provides a packaged solution to capturing data from
      | the FPGA fabric and making it accessible from the CPU.  The block comes in
      | 2 flavors: <i>snap</i> (which captures to a 32 bit wide Shared BRAM), and
      | <i>snap64</i> (which captures to 2x32 bit wide Shared BRAMs to effect a
      | 64 bit capture).
      mask Help: eval('xlWeb(''http://casper.berkeley.edu/wiki/Snap'')')
  time_cntr : xbsIndex_r4/Counter  cnt_type=Free Running  cnt_to=Inf  operation=Up  start_count=0  cnt_by_val=1  arith_type=Unsigned  n_bits=40  bin_pt=0  load_pin=off  rst=on  en=off  explicit_period=on  period=1  dbl_ovrd=off  use_behavioral_HDL=off  implementation=Fabric  block_type=counter
      settings: block_version=11.4
  vacc0 : Subsystem  AncestorBlock=gavrt_library/vacc  mask(vacc){veclen=8, n_inputs=4, max_accum=10, arith_type=0, in_bit_width=32, in_bin_pt=31, out_bit_width=32, out_bin_pt=22, register_din=1, add_latency=2, bram_latency=2, mux_latency=1, use_dsp48=1}
      mask prompts: veclen "Vector Length (2^?)"; n_inputs "Number of Simultaneous Vectors"; max_accum "Maximum # Accumulations (2^?)"; arith_type "Arithmetic Type (0=Unsigned, 1=Signed)"; in_bit_width "Input Bit Width"; in_bin_pt "Input Binary Point"; out_bit_width "Output Bit Width"; out_bin_pt "Output Binary Point"; register_din "Register Input Data  (1 = Enable Register Retiming on input delay)"; add_latency "Add Latency"; bram_latency "BRAM Latency"; mux_latency "Mux Latency"; use_dsp48 "Use DSP48"
      mask help:
      | Sync is expected the clock before the first data to be accumulated.
      | Use the Cram block to feed din for multiple simultaneous inputs.
      | acc_len is the number of vectors to sum.
      | valid is high while a valid accumulation is being clocked out on dout.
      | If only one sync pulse is provided, valid accumulations will repeatedly appear on dout as they become available.
      | Undesired behavior may occur if acc_len is changed without a new sync pulse.
      | Note: The output is an unsigned concatenation of the output streams. Thus, even with only one stream, the output must be recast before using.
      | Register Input Data controls the "Enable Register Retiming" parameter of the delays on 'din'.
      mask init:
      | config.toplevel = gcb;
      | config.source = str2func('vacc_init_xblock');
      | xBlock( config, {...
      |     'veclen', veclen, ...
      |     'n_inputs', n_inputs, ...
      |     'max_accum', max_accum, ...
      |     'arith_type', arith_type, ...
      |     'in_bit_width', in_bit_width, ...
      |     'in_bin_pt', in_bin_pt, ...
      |     'out_bit_width', out_bit_width, ...
      |     'out_bin_pt', out_bin_pt, ...
      |     'register_din', register_din, ...
      |     'add_latency', add_latency, ...
      |     'bram_latency', bram_latency, ...
      |     'mux_latency', mux_latency, ...
      |     'use_dsp48', use_dsp48, ...
      | });
      settings: AttributesFormatString=|
      | vector length=32, inputs=4
      | max accumulations=2^5
  vacc1 : Subsystem  AncestorBlock=gavrt_library/vacc  mask(vacc){veclen=8, n_inputs=4, max_accum=10, arith_type=0, in_bit_width=32, in_bin_pt=31, out_bit_width=32, out_bin_pt=22, register_din=1, add_latency=2, bram_latency=2, mux_latency=1, use_dsp48=1}
      mask prompts: veclen "Vector Length (2^?)"; n_inputs "Number of Simultaneous Vectors"; max_accum "Maximum # Accumulations (2^?)"; arith_type "Arithmetic Type (0=Unsigned, 1=Signed)"; in_bit_width "Input Bit Width"; in_bin_pt "Input Binary Point"; out_bit_width "Output Bit Width"; out_bin_pt "Output Binary Point"; register_din "Register Input Data  (1 = Enable Register Retiming on input delay)"; add_latency "Add Latency"; bram_latency "BRAM Latency"; mux_latency "Mux Latency"; use_dsp48 "Use DSP48"
      mask help:
      | Sync is expected the clock before the first data to be accumulated.
      | Use the Cram block to feed din for multiple simultaneous inputs.
      | acc_len is the number of vectors to sum.
      | valid is high while a valid accumulation is being clocked out on dout.
      | If only one sync pulse is provided, valid accumulations will repeatedly appear on dout as they become available.
      | Undesired behavior may occur if acc_len is changed without a new sync pulse.
      | Note: The output is an unsigned concatenation of the output streams. Thus, even with only one stream, the output must be recast before using.
      | Register Input Data controls the "Enable Register Retiming" parameter of the delays on 'din'.
      mask init: same as ssg_speader_r1/vacc0
      settings: AttributesFormatString=|
      | vector length=32, inputs=4
      | max accumulations=2^5
  vacc2 : Subsystem  AncestorBlock=gavrt_library/vacc  mask(vacc){veclen=8, n_inputs=4, max_accum=10, arith_type=1, in_bit_width=32, in_bin_pt=31, out_bit_width=32, out_bin_pt=22, register_din=1, add_latency=2, bram_latency=2, mux_latency=1, use_dsp48=1}
      mask prompts: veclen "Vector Length (2^?)"; n_inputs "Number of Simultaneous Vectors"; max_accum "Maximum # Accumulations (2^?)"; arith_type "Arithmetic Type (0=Unsigned, 1=Signed)"; in_bit_width "Input Bit Width"; in_bin_pt "Input Binary Point"; out_bit_width "Output Bit Width"; out_bin_pt "Output Binary Point"; register_din "Register Input Data  (1 = Enable Register Retiming on input delay)"; add_latency "Add Latency"; bram_latency "BRAM Latency"; mux_latency "Mux Latency"; use_dsp48 "Use DSP48"
      mask help:
      | Sync is expected the clock before the first data to be accumulated.
      | Use the Cram block to feed din for multiple simultaneous inputs.
      | acc_len is the number of vectors to sum.
      | valid is high while a valid accumulation is being clocked out on dout.
      | If only one sync pulse is provided, valid accumulations will repeatedly appear on dout as they become available.
      | Undesired behavior may occur if acc_len is changed without a new sync pulse.
      | Note: The output is an unsigned concatenation of the output streams. Thus, even with only one stream, the output must be recast before using.
      | Register Input Data controls the "Enable Register Retiming" parameter of the delays on 'din'.
      mask init: same as ssg_speader_r1/vacc0
      settings: AttributesFormatString=|
      | vector length=32, inputs=4
      | max accumulations=2^5
  vacc3 : Subsystem  AncestorBlock=gavrt_library/vacc  mask(vacc){veclen=8, n_inputs=4, max_accum=10, arith_type=1, in_bit_width=32, in_bin_pt=31, out_bit_width=32, out_bin_pt=22, register_din=1, add_latency=2, bram_latency=2, mux_latency=1, use_dsp48=1}
      mask prompts: veclen "Vector Length (2^?)"; n_inputs "Number of Simultaneous Vectors"; max_accum "Maximum # Accumulations (2^?)"; arith_type "Arithmetic Type (0=Unsigned, 1=Signed)"; in_bit_width "Input Bit Width"; in_bin_pt "Input Binary Point"; out_bit_width "Output Bit Width"; out_bin_pt "Output Binary Point"; register_din "Register Input Data  (1 = Enable Register Retiming on input delay)"; add_latency "Add Latency"; bram_latency "BRAM Latency"; mux_latency "Mux Latency"; use_dsp48 "Use DSP48"
      mask help:
      | Sync is expected the clock before the first data to be accumulated.
      | Use the Cram block to feed din for multiple simultaneous inputs.
      | acc_len is the number of vectors to sum.
      | valid is high while a valid accumulation is being clocked out on dout.
      | If only one sync pulse is provided, valid accumulations will repeatedly appear on dout as they become available.
      | Undesired behavior may occur if acc_len is changed without a new sync pulse.
      | Note: The output is an unsigned concatenation of the output streams. Thus, even with only one stream, the output must be recast before using.
      | Register Input Data controls the "Enable Register Retiming" parameter of the delays on 'din'.
      mask init: same as ssg_speader_r1/vacc0
      settings: AttributesFormatString=|
      | vector length=32, inputs=4
      | max accumulations=2^5
  vaccsnap : Subsystem  AncestorBlock=casper_library_scopes/snap64  mask(snap64){nsamples=11}
      mask prompts: nsamples "No. of samples(2^?)"
      mask help:
      | The <i>snap</i> block provides a packaged solution to capturing data from
      | the FPGA fabric and making it accessible from the CPU.  The block comes in
      | 2 flavors: <i>snap</i> (which captures to a 32 bit wide Shared BRAM), and
      | <i>snap64</i> (which captures to 2x32 bit wide Shared BRAMs to effect a
      | 64 bit capture).
      mask Help: eval('xlWeb(''http://casper.berkeley.edu/wiki/Snap'')')
  vaccsynap : Subsystem  AncestorBlock=casper_library_scopes/snap64  mask(snap64){nsamples=11}
      mask prompts: nsamples "No. of samples(2^?)"
      mask help:
      | The <i>snap</i> block provides a packaged solution to capturing data from
      | the FPGA fabric and making it accessible from the CPU.  The block comes in
      | 2 flavors: <i>snap</i> (which captures to a 32 bit wide Shared BRAM), and
      | <i>snap64</i> (which captures to 2x32 bit wide Shared BRAMs to effect a
      | 64 bit capture).
      mask Help: eval('xlWeb(''http://casper.berkeley.edu/wiki/Snap'')')
  wires:
  rst/1 -> Register16/1
  Constant19/1 -> rst/1
  Register16/1 -> Slice2/1
  Slice2/1 -> posedge/1
  posedge/1 -> Delay26/1
  Delay26/1 -> [cnt_rst]
  Constant4/1 -> adc083000x2/4(adc1_data_valid_sim), adc083000x2/3(adc1_sync_sim), adc083000x2/2(adc0_data_valid_sim)
  Constant1/1 -> adc083000x2/1(adc0_sync_sim)
  Slice10/1 -> [adc_sync]
  Register44/1 -> Slice10/1
  adc083000x2/1(adc0_s0) -> [a0]
  adc083000x2/9(adc0_sync) -> Register44/1
  adc083000x2/10(adc0_outofrange) -> Terminator44/1
  adc083000x2/11(adc0_data_valid) -> Terminator45/1
  adc083000x2/12(adc1_s0) -> [b0]
  adc083000x2/20(adc1_sync) -> Terminator43/1
  adc083000x2/21(adc1_outofrange) -> Terminator46/1
  adc083000x2/22(adc1_data_valid) -> Terminator47/1
  Constant20/1 -> adc083000x2/5(sim_adc0_data_in)
  Constant21/1 -> adc083000x2/6(sim_adc1_data_in)
  Concat1/1 -> [default_ip]
  Constant6/1 -> gbe0/7
  gbe0/9 -> Terminator/1
  gbe0/1 -> Terminator17/1
  gbe0/2 -> Terminator16/1
  gbe0/3 -> Terminator15/1
  gbe0/4 -> [txack]
  gbe0/5 -> Terminator8/1
  gbe0/6 -> Terminator6/1
  gbe0/7 -> Terminator5/1
  gbe0/8 -> Terminator3/1
  gbe0/10 -> Terminator11/1
  Constant5/1 -> gbe0/8
  Delay21/1 -> gbe0/6
  Delay22/1 -> gbe0/5
  Delay24/1 -> gbe0/4
  Delay25/1 -> gbe0/3
  Delay29/1 -> gbe0/2
  Delay30/1 -> gbe0/1
  Constant25/1 -> Mux4/2
  Mux4/1 -> Register22/1
  acc_len/1 -> Mux4/3
  acc_len_sel/1 -> Slice1/1
  Constant26/1 -> acc_len/1
  Register22/1 -> [acc_len]
  Constant3/1 -> acc_len_sel/1
  posedge7/1 -> [anew_acc]
  Slice1/1 -> Mux4/1
  Constant29/1 -> fftshift/1
  fftshift/1 -> Delay53/1
  Delay53/1 -> [fftshift]
  adc083000x2/16(adc1_s4) -> [b4]
  adc083000x2/13(adc1_s1) -> [b1]
  adc083000x2/15(adc1_s3) -> [b3]
  adc083000x2/17(adc1_s5) -> [b5]
  adc083000x2/19(adc1_s7) -> [b7]
  adc083000x2/3(adc0_s2) -> [a2]
  adc083000x2/5(adc0_s4) -> [a4]
  adc083000x2/7(adc0_s6) -> [a6]
  adc083000x2/2(adc0_s1) -> [a1]
  adc083000x2/4(adc0_s3) -> [a3]
  adc083000x2/6(adc0_s5) -> [a5]
  adc083000x2/8(adc0_s7) -> [a7]
  adc083000x2/14(adc1_s2) -> [b2]
  adc083000x2/18(adc1_s6) -> [b6]
  err_clear_sim1/1 -> dest_ip/1
  dest_ip/1 -> [ip_addr]
  dest_port/1 -> Slice7/1
  err_clear_sim3/1 -> dest_port/1
  Slice7/1 -> [port]
  Constant/1 -> Concat1/1
  Constant7/1 -> Concat1/2
  Constant8/1 -> Concat1/3
  Constant9/1 -> Concat1/4
  [default_ip] -> Mux/2
  [ip_addr] -> Mux/3
  err_clear_sim2/1 -> ip_select/1
  ip_select/1 -> Slice8/1
  Slice8/1 -> [ip_select]
  [ip_select] -> Mux/1
  Constant10/1 -> Mux1/2
  [port] -> Mux1/3
  [port_select] -> Mux1/1
  err_clear_sim4/1 -> port_select/1
  port_select/1 -> Slice9/1
  Slice9/1 -> [port_select]
  Mux1/1 -> [dest_port]
  Mux/1 -> [dest_ip]
  Delay1/1 -> [sync_out]
  vacc0/1(valid) -> [valid], posedge7/1
  [cnt_rst] -> Delay30/1
  [data_out] -> speader/1(data_in)
  [data_valid] -> speader/2(valid_in)
  [dest_ip] -> Delay24/1
  [dest_port] -> Delay22/1
  speader/3(eof) -> Delay50/1
  [eof] -> Delay21/1
  Constant18/1 -> speader/3(heap_size)
  Constant33/1 -> speader/8(mode)
  Constant34/1 -> speader/10(payload_offset)
  speader/2(data_valid) -> Delay35/1
  [data_valid_spead] -> Delay25/1
  [data_spead] -> Delay29/1
  heap_cntr/1 -> [heap_cnt]
  Gateway Out10/1 -> Scope8/1
  Gateway Out11/1 -> Scope8/2
  Gateway Out13/1 -> Scope8/3
  [eof] -> Gateway Out11/1
  [data_valid_spead] -> Gateway Out10/1
  [data_spead] -> Gateway Out13/1
  Delay35/1 -> [data_valid_spead]
  [cnt_rst] -> time_cntr/1
  Delay44/1 -> [data_spead]
  [not_blank_num] -> Convert/1
  Constant24/1 -> speader/4(Packet_length)
  [cnt_rst] -> spectrum_cntr/1
  [eoh] -> spectrum_cntr/2
  [cnt_rst] -> speader/11(Reset)
  Convert/1 -> speader/7(integration size)
  speader/1(data_out) -> Delay44/1
  [sync_gen] -> Delay1/1
  spectrum_cntr/1 -> [spec_cntr]
  time_cntr/1 -> [time_cntr]
  [time_cntr] -> speader/5(time_stamp)
  [spec_cntr] -> speader/6(spectrum counter)
  [xxout0_1] -> vacc0/3(din_1_1)
  [xxout1_1] -> vacc0/4(din_2_1)
  [xxout2_1] -> vacc0/5(din_3_1)
  [xxout3_1] -> vacc0/6(din_4_1)
  [yyout0_1] -> vacc1/3(din_1_1)
  [yyout1_1] -> vacc1/4(din_2_1)
  [yyout2_1] -> vacc1/5(din_3_1)
  [yyout3_1] -> vacc1/6(din_4_1)
  [xyoutre0_1] -> vacc2/3(din_1_1)
  [xyoutre1_1] -> vacc2/4(din_2_1)
  [xyoutre2_1] -> vacc2/5(din_3_1)
  [xyoutre3_1] -> vacc2/6(din_4_1)
  [xyoutim0_1] -> vacc3/3(din_1_1)
  [xyoutim1_1] -> vacc3/4(din_2_1)
  [xyoutim2_1] -> vacc3/5(din_3_1)
  [xyoutim3_1] -> vacc3/6(din_4_1)
  cram4/1(Out) -> [din]
  vacc0/2(dout_1_1) -> [xx_vacc0]
  vacc0/3(dout_2_1) -> [xx_vacc1]
  vacc1/2(dout_1_1) -> [yy_vacc0]
  vacc1/3(dout_2_1) -> [yy_vacc1]
  vacc2/2(dout_1_1) -> [xy_vaccre0]
  vacc2/3(dout_2_1) -> [xy_vaccre1]
  vacc3/2(dout_1_1) -> [xy_vaccim0]
  vacc3/3(dout_2_1) -> [xy_vaccim1]
  vacc0/4(dout_3_1) -> [xx_vacc2]
  vacc0/5(dout_4_1) -> [xx_vacc3]
  vacc2/4(dout_3_1) -> [xy_vaccre2]
  vacc2/5(dout_4_1) -> [xy_vaccre3]
  vacc3/4(dout_3_1) -> [xy_vaccim2]
  vacc3/5(dout_4_1) -> [xy_vaccim3]
  [xx_vacc0] -> cram4/1(In1)
  [yy_vacc0] -> cram4/2(In2)
  [xy_vaccre0] -> cram4/3(In3)
  [xy_vaccim0] -> cram4/4(In4)
  [xx_vacc1] -> cram4/5(In5)
  [yy_vacc1] -> cram4/6(In6)
  [xy_vaccre1] -> cram4/7(In7)
  [xy_vaccim1] -> cram4/8(In8)
  [xx_vacc2] -> cram4/9(In9)
  [yy_vacc2] -> cram4/10(In10)
  [xy_vaccre2] -> cram4/11(In11)
  [xy_vaccim2] -> cram4/12(In12)
  [xx_vacc3] -> cram4/13(In13)
  [yy_vacc3] -> cram4/14(In14)
  [xy_vaccre3] -> cram4/15(In15)
  [xy_vaccim3] -> cram4/16(In16)
  Delay50/1 -> [eof]
  [cnt_rst] -> heap_cntr/1
  [eof] -> heap_cntr/2
  speader/4(eoh) -> Delay3/1
  Delay3/1 -> [eoh]
  [sync_out] -> vacc0/1(sync)
  [acc_len] -> vacc0/2(acc_len)
  [acc_len] -> vacc3/2(acc_len)
  [sync_out] -> vacc1/1(sync)
  [sync_out] -> vacc2/1(sync)
  [sync_out] -> vacc3/1(sync)
  [acc_len] -> vacc2/2(acc_len)
  [acc_len] -> vacc1/2(acc_len)
  vacc1/1(valid) -> Terminator1/1
  vacc2/1(valid) -> Terminator4/1
  vacc3/1(valid) -> Terminator7/1
  vacc1/4(dout_3_1) -> [yy_vacc2]
  vacc1/5(dout_4_1) -> [yy_vacc3]
  reshaper/2(sel) -> Terminator10/1
  reshaper/3(header_valid_out) -> Terminator13/1
  negedge2/1 -> reshaper/1(rst)
  [din] -> Delay13/1
  Delay10/1 -> Delay11/1, negedge2/1
  Delay13/1 -> Delay12/1
  Delay12/1 -> reshaper/3(din)
  Delay11/1 -> reshaper/2(valid)
  reshaper/5(st) -> Terminator14/1
  Delay14/1 -> [data_out]
  Delay15/1 -> [data_valid]
  reshaper/1(dout) -> Delay14/1
  reshaper/4(data_valid_out) -> Delay15/1
  Constant11/1 -> length/1
  Constant27/1 -> ssg_bram/2(data_in)
  Constant28/1 -> ssg_bram/3(we)
  length/1 -> cycle_limit/2(cnt_limit)
  dur_len/1(at_limit) -> Counter/2
  cycle_limit/1(at_limit) -> Counter/1
  Counter/1 -> ssg_bram/1(addr)
  ssg_bram/1(data_out) -> SuperSlice/1(In)
  SuperSlice/1(DUR) -> [DUR]
  SuperSlice/2(AS/R) -> [ASR]
  SuperSlice/3(S/R1) -> [SR1]
  SuperSlice/4(S/R0) -> [SR0]
  SuperSlice/5(CAL) -> [CAL]
  SuperSlice/6(BLANK) -> [LOC_BLANK]
  Constant30/1 -> Register19/1
  Register18/1 -> Inverter/1
  Inverter/1 -> Register19/2  "ppsready"
  Constant31/1 -> Register18/1
  sg/1(sync_out) -> [sync_gen]
  sg/2(pps_out) -> [master_rst]
  arm/1 -> Register20/1
  Constant12/1 -> arm/1
  Register20/1 -> Slice3/1
  Slice3/1 -> [arm]
  [arm] -> Register18/2
  [master_rst] -> Register18/3
  [sync_out] -> Register19/3
  Register19/1 -> [data_enable]
  [valid] -> Logical/1
  [data_enable] -> Logical/2
  Logical/1 -> Delay10/1, negedge1/1
  [a0] -> cram/1(In1)
  [a1] -> cram/2(In2)
  [a2] -> cram/3(In3)
  [a3] -> cram/4(In4)
  [a4] -> cram/5(In5)
  [a5] -> cram/6(In6)
  [a6] -> cram/7(In7)
  [a7] -> cram/8(In8)
  cram/1(Out) -> adcsnap/1(din)
  Constant14/1 -> adcsnap/3(we), adcsnap/2(trig)
  cram3/1(Out) -> vaccsnap/1(din)
  [xx_vacc0] -> cram3/1(In1)
  [xx_vacc1] -> cram3/2(In2)
  [anew_acc] -> vaccsnap/2(trig)
  [valid] -> vaccsnap/3(we)
  [data_spead] -> Delay2/1
  [data_valid_spead] -> pktsnap/3(we)
  [eoh] -> pktsnap/2(trig)
  Delay2/1 -> pktsnap/1(din)
  [data_valid] -> bus_create/2(in2)
  [data_valid_spead] -> bus_create/3(in3)
  [eof] -> bus_create/4(in4)
  [cnt_rst] -> bus_create/5(in5)
  [arm] -> bus_create/6(in6)
  [master_rst] -> bus_create/7(in7)
  [sync_out] -> bus_create/8(in8)
  [data_enable] -> bus_create/9(in9)
  [valid] -> bus_create/10(in10)
  [sync_gen] -> stat/2(trig)
  [data_valid_spead] -> stat/3(we)
  [txack] -> bus_create/1(in1)
  bus_create1/1(bus_out) -> stat/1(din)
  Constant16/1 -> bus_create1/1(in1)
  bus_create/1(bus_out) -> bus_create1/2(in2)
  [status_bits] -> Delay4/1
  Delay4/1 -> Convert1/1
  cram5/1(Out) -> vaccsynap/1(din)
  [yy_vacc0] -> cram5/1(In1)
  [yy_vacc1] -> cram5/2(In2)
  [anew_acc] -> vaccsynap/2(trig)
  [valid] -> vaccsynap/3(we)
  [adc_sync] -> sg/1(pps)
  Constant13/1 -> [xxout0], [yyout0], [xyoutre0], [xyoutim0], [xxout1], [yyout1], [xyoutre1], [xyoutim1], [xxout2], [yyout2], [xyoutre2], [xyoutim2], [xxout3], [yyout3], [xyoutre3], [xyoutim3]
  [xxout0] -> bus_create3/1(in1)
  [xxout1] -> bus_create3/2(in2)
  [xxout2] -> bus_create3/3(in3)
  [xxout3] -> bus_create3/4(in4)
  [yyout0] -> bus_create3/5(in5)
  [yyout1] -> bus_create3/6(in6)
  [yyout2] -> bus_create3/7(in7)
  [yyout3] -> bus_create3/8(in8)
  [xyoutre0] -> bus_create3/9(in9)
  [xyoutre1] -> bus_create3/10(in10)
  [xyoutre2] -> bus_create3/11(in11)
  [xyoutre3] -> bus_create3/12(in12)
  [xyoutim0] -> bus_create3/13(in13)
  [xyoutim1] -> bus_create3/14(in14)
  [xyoutim2] -> bus_create3/15(in15)
  [xyoutim3] -> bus_create3/16(in16)
  Constant2/1 -> Mux2/3
  bus_create3/1(bus_out) -> Mux2/2
  Mux2/1 -> bus_expand/1(bus_in)
  bus_expand/2(lsb_out1) -> bus_expand2/1(bus_in)
  bus_expand/1(msb_out2) -> bus_expand1/1(bus_in)
  bus_expand1/1(msb_out8) -> [xxout0_1]
  bus_expand1/2(out7) -> [yyout0_1]
  bus_expand1/3(out6) -> [xyoutre0_1]
  bus_expand1/4(out5) -> [xyoutim0_1]
  bus_expand1/5(out4) -> [xxout1_1]
  bus_expand1/6(out3) -> [yyout1_1]
  bus_expand1/7(out2) -> [xyoutre1_1]
  bus_expand1/8(lsb_out1) -> [xyoutim1_1]
  bus_expand2/1(msb_out8) -> [xxout2_1]
  bus_expand2/2(out7) -> [yyout2_1]
  bus_expand2/3(out6) -> [xyoutre2_1]
  bus_expand2/4(out5) -> [xyoutim2_1]
  bus_expand2/5(out4) -> [xxout3_1]
  bus_expand2/6(out3) -> [yyout3_1]
  bus_expand2/7(out2) -> [xyoutre3_1]
  bus_expand2/8(lsb_out1) -> [xyoutim3_1]
  Constant22/1 -> Mux2/1
  negedge1/1 -> [int_tick]
  [master_rst] -> Counter1/1
  Counter1/1 -> Slice5/1, Slice4/1
  Slice5/1 -> negedge/1
  Slice4/1 -> [spec_cnt]
  negedge/1 -> [spec_tick]
  [spec_tick] -> cycle_limit/1(cnt_en), dur_len/1(cnt_en)
  [DUR] -> dur_len/2(cnt_limit)
  [master_rst] -> dur_len/3(master_rst)
  [master_rst] -> cycle_limit/3(master_rst)
  [SR0] -> bus_create4/4(in4)
  [SR0] -> bus_create4/3(in3)
  [CAL] -> bus_create4/2(in2)
  [LOC_BLANK] -> bus_create4/1(in1)
  bus_create4/1(bus_out) -> Register1/1
  Register1/1 -> bus_expand3/1(bus_in), Mux3/2
  bus_expand3/2(out3) -> leds_gpios/1(IN0)
  bus_expand3/3(out2) -> leds_gpios/2(IN1)
  bus_expand3/4(lsb_out1) -> leds_gpios/3(IN2)
  err_clear_sim5/1 -> gpio/1
  gpio/1 -> Register2/1
  [spec_tick] -> Register2/2
  Register2/1 -> Mux3/3
  err_clear_sim6/1 -> master_slave_sel/1
  Slice/1 -> Mux3/1
  master_slave_sel/1 -> Slice/1
  Mux3/1 -> Slice6/1, Register3/1
  Slice6/1 -> [blank]
  [int_tick] -> Register3/2
  Register3/1 -> [status_bits]
  [blank] -> Inverter1/1
  [spec_tick] -> Logical1/2
  Logical1/1 -> number_of_good_spectra/2
  Delay/1 -> number_of_good_spectra/1
  number_of_good_spectra/1 -> Register/1
  [int_tick] -> Delay/1
  [int_tick] -> Register/2
  Register/1 -> [not_blank_num]
  Inverter1/1 -> Logical1/1
  Convert1/1 -> speader/9(status_bits)
